simulink model "sim1"  (R2023b)
settings: Solver=VariableStepAuto  StartTime=0.0  StopTime=200  RelTol=1e-3
model workspace (MAT data in the model file):
  c = Simulink.Parameter
  c.Value = 0.1
  c.DataType = 'auto'
  c.DocUnits = 'Ns/m^3'
  c.Complexity = 'real'
  c.Dimensions = [1 1]
  k = Simulink.Parameter
  k.Value = 0.1
  k.DataType = 'auto'
  k.DocUnits = '<N/m>'
  k.Complexity = 'real'
  k.Dimensions = [1 1]
  m = Simulink.Parameter
  m.Value = 1
  m.DataType = 'auto'
  m.DocUnits = 'kg'
  m.Complexity = 'real'
  m.Dimensions = [1 1]
settings Model: Creator=anura  LastModifiedBy=anura
settings DataIOCC: ReturnWorkspaceOutputs=off

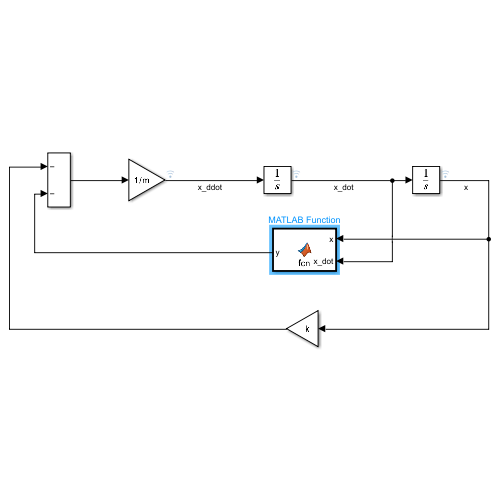
[thumbnail: Simulink's stored preview of the top-level diagram]
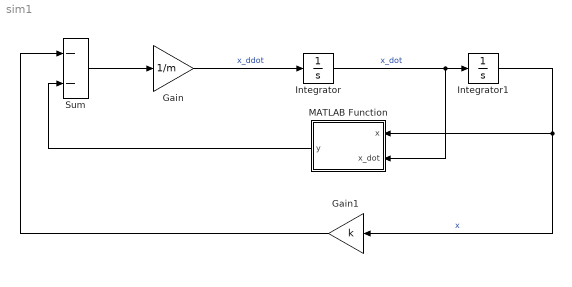
== system sim1 ==
  Gain : Gain  Gain=1/m
  Gain1 : Gain  Gain=k
  Integrator : Integrator  InitialCondition=-1
  Integrator1 : Integrator  InitialCondition=3
  MATLAB Function : MATLAB Function  TreatAsAtomicUnit=on
  Sum : Sum  Inputs=--
  wires:
  Gain/1 -> Integrator/1  "x_ddot"
  Integrator/1 -> MATLAB Function/2(x_dot), Integrator1/1  "x_dot"
  Sum/1 -> Gain/1
  Integrator1/1 -> MATLAB Function/1(x), Gain1/1  "x"
  Gain1/1 -> Sum/1
  MATLAB Function/1(y) -> Sum/2

== matlab function sim1/MATLAB Function ==
  data: x input; y output; x_dot input
function y = fcn(x, x_dot)
    c = 0.1;
    y = 2*c*(x^2 - 1)*x_dot;
end
